simulink subsystem "Model_LAB4_controller_nomtracking"  (R2024b)
settings: Solver=VariableStepAuto  StartTime=0.0  StopTime=10.0  RelTol=1e-3
values from neighbouring files (symbols this model uses):
  K_i = 0    [A_final_results.m]
  Nu = Sol(5,:)    [A_final_results.m]
  Nx = Sol(1:4,:)    [A_final_results.m]
undefined symbols (not defined in the file or in its folder): DiscIntNeverNeededParam, drv, K_fb
settings Model: Creator=Utente  LastModifiedBy=Buton

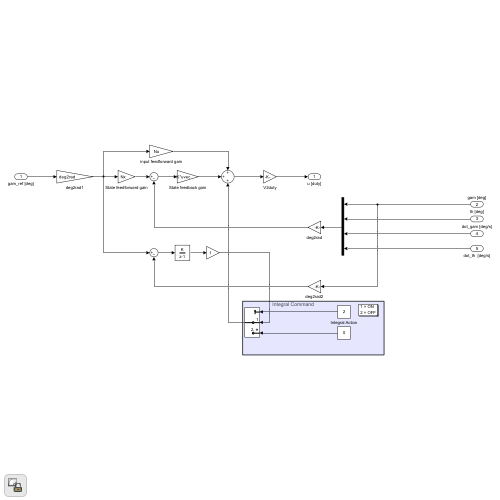
[thumbnail: Simulink's stored preview of the top-level diagram]
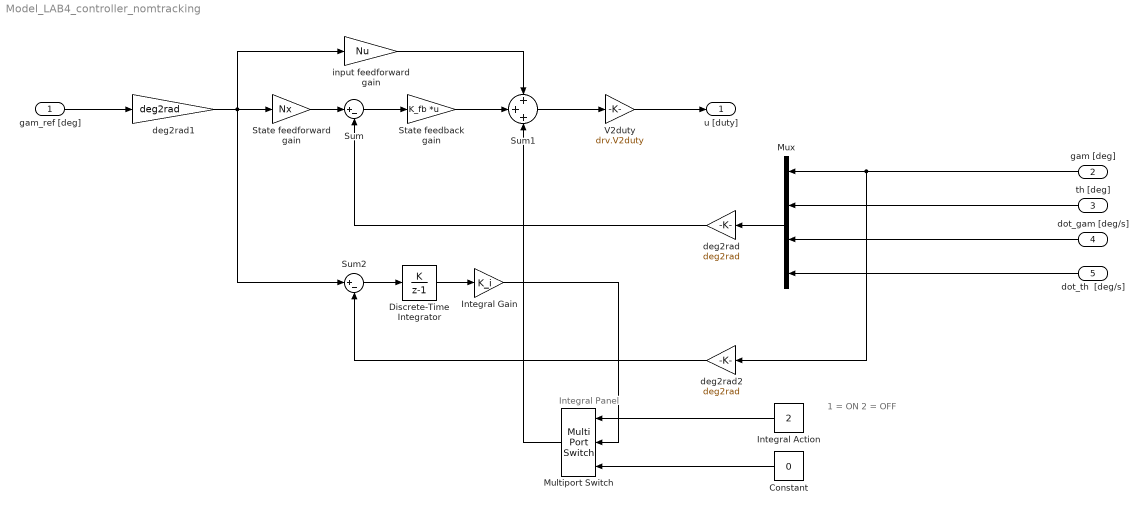
== system Model_LAB4_controller_nomtracking ==
  note: Integral Panel
  note: 1 = ON
      | 2 = OFF
  gam_ref [deg] : Inport
  gam [deg] : Inport  Port=2
  th [deg] : Inport  Port=3
  dot_gam [deg/s] : Inport  Port=4
  dot_th  [deg/s] : Inport  Port=5
  Constant : Constant  Value=0
  Discrete-Time Integrator : DiscreteIntegrator  IntegratorMethod=Accumulation: Forward Euler  SampleTime=-1  ICPrevOutput=DiscIntNeverNeededParam  ICPrevScaledInput=DiscIntNeverNeededParam
  Integral Action : Constant  Value=2
  Integral Gain : Gain  Gain=K_i
  Multiport Switch : MultiPortSwitch  Inputs=2  SaturateOnIntegerOverflow=off  InputSameDT=off
  Mux : Mux
  State feedback gain : Gain  Gain=K_fb  Multiplication=Matrix(K*u) (u vector)
  State feedforward gain : Gain  Gain=Nx
  Sum : Sum  Inputs=|+-
  Sum1 : Sum  Inputs=+++
  Sum2 : Sum  Inputs=|+-
  V2duty : Gain  Gain=drv.V2duty
  deg2rad : Gain  Gain=deg2rad
  deg2rad1 : Gain  Gain=deg2rad
  deg2rad2 : Gain  Gain=deg2rad
  input feedforward gain : Gain  Gain=Nu
  u [duty] : Outport
  wires:
  dot_th  [deg/s]/1 -> Mux/4
  State feedback gain/1 -> Sum1/2
  gam [deg]/1 -> Mux/1, deg2rad2/1
  th [deg]/1 -> Mux/2
  gam_ref [deg]/1 -> deg2rad1/1
  State feedforward gain/1 -> Sum/1
  Sum1/1 -> V2duty/1
  Sum/1 -> State feedback gain/1
  input feedforward gain/1 -> Sum1/1
  deg2rad1/1 -> input feedforward gain/1, State feedforward gain/1, Sum2/1
  dot_gam [deg/s]/1 -> Mux/3
  V2duty/1 -> u [duty]/1
  Mux/1 -> deg2rad/1
  deg2rad/1 -> Sum/2
  deg2rad2/1 -> Sum2/2
  Sum2/1 -> Discrete-Time Integrator/1
  Discrete-Time Integrator/1 -> Integral Gain/1
  Constant/1 -> Multiport Switch/3
  Multiport Switch/1 -> Sum1/3
  Integral Gain/1 -> Multiport Switch/2
  Integral Action/1 -> Multiport Switch/1
